simulink model "ES002A_McuDiagc"  (R2013b)
settings: Solver=FixedStepDiscrete  SolverMode=SingleTasking  StartTime=0.0  StopTime=1  FixedStep=0.000125  RelTol=1e-3
values from neighbouring files (symbols this model uses):
  dMcuDiagcFastLoopCntrMax = DataDict.Display    [ES002A_McuDiagc_DataDict.m]
  dMcuDiagcFastLoopCntrMin = DataDict.Display    [ES002A_McuDiagc_DataDict.m]
  dMcuDiagcLoopCntr2MilliSecMotCtrlDif = DataDict.Display    [ES002A_McuDiagc_DataDict.m]
  FastLoopCntr = DataDict.IpSignal    [ES002A_McuDiagc_DataDict.m]
  FASTLOOPCNTRMAX_CNT_U08 = DataDict.Constant    [ES002A_McuDiagc_DataDict.m]
  FASTLOOPCNTRMIN_CNT_U08 = DataDict.Constant    [ES002A_McuDiagc_DataDict.m]
  FastLoopCntrPrev = DataDict.PIM    [ES002A_McuDiagc_DataDict.m]
  LOOPCNTR2MILLISECMOTCTRLCOMPPRM_CNT_U08 = DataDict.Constant    [ES002A_McuDiagc_DataDict.m]
  LOSSMOTCTRLLOOPPRM_CNT_U08 = DataDict.Constant    [ES002A_McuDiagc_DataDict.m]
  McuDiagc2MilliSecCntrCompThd = DataDict.Calibration    [ES002A_McuDiagc_DataDict.m]
  McuDiagcFlt = DataDict.NTC    [ES002A_McuDiagc_DataDict.m]
  McuDiagcFltFailStep = DataDict.Calibration    [ES002A_McuDiagc_DataDict.m]
  McuDiagcFltPassStep = DataDict.Calibration    [ES002A_McuDiagc_DataDict.m]
  MOTCTRLDIAGCINITDLY_CNT_U08 = DataDict.Constant    [ES002A_McuDiagc_DataDict.m]
undefined symbols (not defined in the file or in its folder): NtcSts1, sigbuilder_block
libraries: simulink x10, NxtrMax x1, NxtrMin x1
(part 1 of 2)
settings Model: RequirementInfo="{}  %GIDa_ca294f38_ed7c_4fb9_8c54_f4d56271bfc7"  ModifiedHistory=Rev 008: Updated model to Matlab 2013B, added comments to show requirement linkage  Creator=nz3zln  LastModifiedBy=wzvp6q
settings SolverCC: AutoInsertRateTranBlk=on  InsertRTBMode=Always
settings DataIOCC: LimitDataPoints=off  SaveFormat=Structure  ReturnWorkspaceOutputs=on
settings OptimizationCC: BlockReduction=off  InlineParams=on  ZeroExternalMemoryAtStartup=off  ZeroInternalMemoryAtStartup=off  OptimizeModelRefInitCode=on  LifeSpan=1
settings DebuggingCC: SignalInfNanChecking=error  SignalRangeChecking=warning  UnderspecifiedInitializationDetection=Simplified  SolverPrmCheckMsg=error  InheritedTsInSrcMsg=error  DiscreteInheritContinuousMsg=error  SingleTaskRateTransMsg=error  TasksWithSamePriorityMsg=error  SigSpecEnsureSampleTimeMsg=error  CheckMatrixSingularityMsg=error  ParameterUnderflowMsg=error  ParameterPrecisionLossMsg=error  ParameterTunabilityLossMsg=error  FixptConstUnderflowMsg=warning  FixptConstOverflowMsg=warning  VectorMatrixConversionMsg=error  SignalLabelMismatchMsg=error  UnconnectedInputMsg=error  UnconnectedOutputMsg=error  UnconnectedLineMsg=error  SFcnCompatibilityMsg=error  UniqueDataStoreMsg=warning  BusObjectLabelMismatch=error  RootOutportRequireBusObject=error  AssertControl=DisableAll  ModelReferenceIOMsg=error  ModelReferenceVersionMismatchMessage=warning  ModelReferenceIOMismatchMessage=error  ModelReferenceCSMismatchMessage=warning  ModelReferenceDataLoggingMessage=error  StateNameClashWarn=warning  StrictBusMsg=ErrorOnBusTreatedAsVector  NonBusSignalsTreatedAsBus=error  SFUnexpectedBacktrackingDiag=error  SFInvalidInputDataAccessInChartInitDiag=error  SFNoUnconditionalDefaultTransitionDiag=error  SFTransitionOutsideNaturalParentDiag=error  SFUnconditionalTransitionShadowingDiag=error  SFUndirectedBroadcastEventsDiag=error
settings ModelReferenceCC: ModelReferenceNumInstancesAllowed=Single
settings RTWCC: SystemTargetFile=autosar.tlc  GenCodeOnly=on  TemplateMakefile=ert_default_tmf  Description=AUTOSAR  GenerateReport=on  ProcessScript=autosar_make_rtw_hook  LaunchReport=on
settings CodeAppCC: GenerateComments=off  IgnoreCustomStorageClasses=off  CustomSymbolStrType=$N$R$M  CustomSymbolStrBlkIO=$N$M  SimulinkBlockComments=off
settings STFCustomTargetCC: ParMdlRefBuildCompliant=on  CompOptLevelCompliant=on  IncludeMdlTerminateFcn=off  CombineOutputUpdateFcns=on  SuppressErrorStatus=on  ERTFirstTimeCompliant=on  ERTCustomFileBanners=on  SupportNonFinite=off  SupportComplex=off  SupportContinuousTime=off  SupportNonInlinedSFcns=off  MATLABClassNameForMDSCustomization=Simulink.SoftwareTarget.ERTCustomization  AutosarCompliant=on  GRTInterface=off  SystemTargetFile=autosar.tlc
settings ERTTargetCC: CodeReplacementLibrary=ANSI_C  ConcurrentExecutionCompliant=off  IncludeMdlTerminateFcn=off  SuppressErrorStatus=on  SupportNonFinite=off  SupportComplex=off  ModelStepFunctionPrototypeControlCompliant=off  CPPClassGenCompliant=off  AutosarCompliant=on  InlinedParameterPlacement=NonHierarchical  ERTCustomFileTemplate=example_file_process.tlc  EnableUserReplacementTypes=on

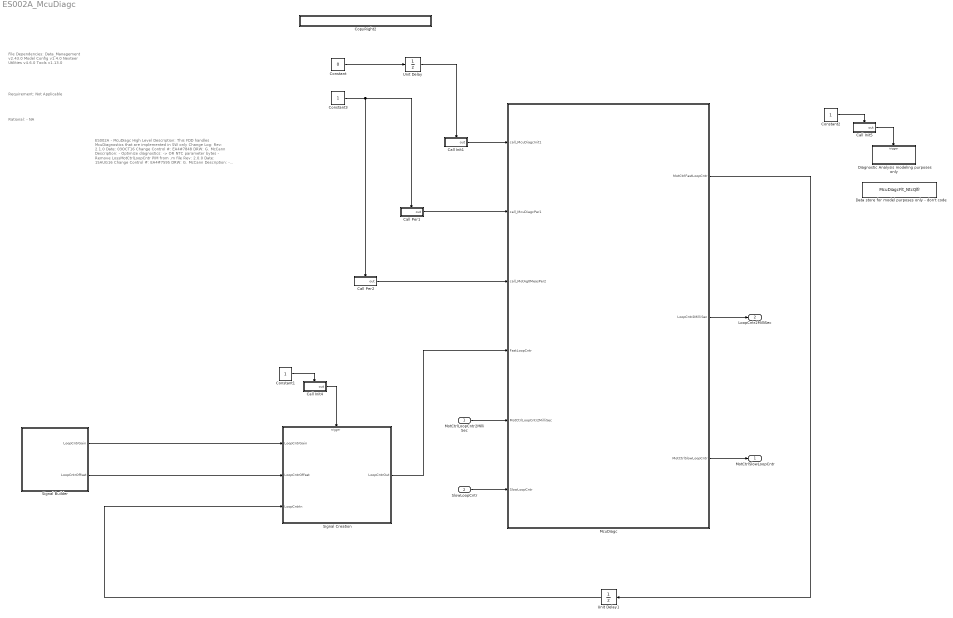
== system ES002A_McuDiagc ==
  note: ES002A - McuDiagc
      | High Level Description:
      | This FDD handles McuDiagnostics that are implemented in SW only
      |
      | Change Log:
      |
      | Rev: 2.1.0
      | Date: 03OCT16
      | Change Control #: EA4#7848
      | DRW: G. McCann
      | Description:
      | - Optimize diagnostics:
      |    -> OR NTC parameter bytes
      | - Remove LossMotCtrlLoopCntr PIM from .m file
      |
      | Rev: 2.0.0
      | Date: 15AUG16
      | Change Control #: EA4#7595
      | DRW: G. McCann
      | Description:
      | - Optimize diagnostics:
      |    -> Remove Per3 and associated IRVs
      |    -> Move relevant diagnostics that were in Per3 to Per2
      | - M file change: Update "ReadIn" property of input signals
      | "MotCtrlLoopCntr2MilliSec" and "SlowLoopCntr"
      |
      | Rev: 1.5.0
      | Date: 28JUN16
      | Change Control #: ICR-EA4#6452
      | DRW: G. McCann
      | Description:
      | -  Add IRVs for passing FastLoopCntrDiagcCfgd from Per2 to Per3.
      | This will allow a constant number of 2ms loops to pass before doing
      | the initial fault determination in Per3.
      | - Add IRV to pass LossMotCtrlLoopCntr from Per2 to Per3.  This
      | corrects an issue with the previous revision in which the same PIM
      | was being used in two different periodic functions.
      |
      | Rev: 1.4.0
      | Date: 15JUN16
      | Change Control #: ICR-EA4#6157
      | DRW: G. McCann
      | Description:
      | -  Add diagnostic check to ensure the MotCtrl ISR is
      | receiving information from the 2ms periodic.
      |
      | Rev: 1.3.0
      | Date: 07JUN16
      | Change Control #: ICR-EA4#6089
      | DRW: K. Patel
      | Description:
      | - ISO Debounce logic Added for NTC 2B
      |
      | Rev: 1.2.0
      | Date: 09MAY16
      | Change Control #: ICR-EA4#5733
      | DRW: G. McCann
      | Description:
      | - Add conditional to McuDiagcPer2 to allow a constant number
      | of 2ms loops to pass before doing the initial fault determination
      |
      | Rev: 1.0.0
      | Date: 23MAR16
      | Change Control #: ICR-EA4#49112
      | DRW: J. Erlenbeck
      | Description:
      | - Initial Release
  note: File Dependencies:
      | Data_Management v2.43.0
      | Model Config v1.4.0
      | Nexteer Utilities v4.6.0
      | Tools v1.13.0
  note: Requirement:
      | Not Applicable
  note: Rational:
      | - NA
  MotCtrlLoopCntr2MilliSec : Inport  RequirementInfo={} %GIDa_ea001b4b_5ccc_4bc9_bc0a_5435325e31ab  OutDataTypeStr=uint16
  SlowLoopCntr : Inport  Port=2  OutDataTypeStr=uint16
  Call Init1 : Subsystem  TreatAsAtomicUnit=on
  Call Init4 : Subsystem  TreatAsAtomicUnit=on
  Call Init5 : Subsystem  TreatAsAtomicUnit=on
  Call Per1 : Subsystem  TreatAsAtomicUnit=on
  Call Per2 : Subsystem  TreatAsAtomicUnit=on
  Constant : Constant  Value=0  OutDataTypeStr=uint8
  Constant1 : Constant  OutDataTypeStr=int8
  Constant2 : Constant  OutDataTypeStr=int8
  Constant3 : Constant  OutDataTypeStr=int8
  CopyRight2 : Subsystem  Description=|  mask(Copyright Information){none=on}
      | Copyright info block.                                               
      |                                                                     
      | Place copyright information at the top of every subsystem in design.
      mask prompts: none "No parameters"
      mask help: Place copyright information at the top of every subsystem in design.
      mask Display:
      | NxtrConf = 'Nexteer Confidential';
      | 
      | sys = bdroot; %handle for the current model ("system")
      | first = get_param(sys,'Created');
      | first = first(end-3:end);  %year is last four digits
      | 
      | last = get_param(sys,'LastModifiedDate');
      | if isempty(last)
      |     last = datestr(now,'yyyy');
      | else
      |     last = last(end-3:end);
      | end
      | 
      | if strcmp(first,last)
      |     fprintf('%s -- Copyright %s Nexteer',NxtrConf,first)
      | else
      |     fprintf('%s -- %s%s- %s Nexteer',NxtrConf,char(169),first,last)
      | end
  Data store for model purposes only - don't code : DataStoreMemory  DataStoreName=McuDiagcFlt_NtcQlfr
  Diagnostic Analysis modeling purposes only : Subsystem  TreatAsAtomicUnit=on
  McuDiagc : Subsystem
  Signal Builder : Subsystem  Tag=STV Subsys  LoadFcn=sigbuilder_block('load');  StartFcn=sigbuilder_block('start');  StopFcn=sigbuilder_block('stop');  ClipboardFcn=sigbuilder_block('clipboard');  mask(Sigbuilder block){}
      mask help: Simulink:masks:SigbuilderBlock_MD
      mask init:
      | if ~strcmp(get_param(bdroot(gcbh),'SimulationStatus'),'stopped') tuvar = sigbuilder_block('maskInit'); end
      settings: CopyFcn=sigbuilder_block('copy');  DeleteFcn=sigbuilder_block('delete');  ModelCloseFcn=sigbuilder_block('modelClose');  PreSaveFcn=sigbuilder_block('preSave');  PauseFcn=sigbuilder_block('pause');  ContinueFcn=sigbuilder_block('continue');  NameChangeFcn=sigbuilder_block('namechange');  OpenFcn=sigbuilder_block('open',[6 6 1012.5 507 ]);  CloseFcn=sigbuilder_block('close');
      mask Display: plot(0, 0, 100, 100,[2, 2, 32, 32, 2], [68, 8, 8, 68, 68],[32, 2], [38, 38], [32, 19, 2],[53, 60, 44], [32, 17, 17, 2],[16, 16, 31, 31]);txt = getActiveGroup(gcbh);text(2, 100, txt,'verticalAlignment', 'top');
  Signal Creation : Subsystem
  Unit Delay : UnitDelay  InitialCondition=1  SampleTime=-1
  Unit Delay1 : UnitDelay  SampleTime=-1
  MotCtrlSlowLoopCntr : Outport
  LoopCntr2MilliSec : Outport  Port=2
  wires:
  Constant/1 -> Unit Delay/1
  Unit Delay/1 -> Call Init1/Enable
  Constant3/1 -> Call Per1/Enable, Call Per2/Enable
  Call Init1/1(out) -> McuDiagc/1(call_McuDiagcInit1)
  Call Per1/1(out) -> McuDiagc/2(call_McuDiagcPer1)
  Call Per2/1(out) -> McuDiagc/3(call_MotAg0MeasPer2)
  Unit Delay1/1 -> Signal Creation/3(LoopCntrIn)
  Constant1/1 -> Call Init4/Enable
  Call Init4/1(out) -> Signal Creation/Trigger
  Signal Builder/1(LoopCntrGain) -> Signal Creation/1(LoopCntrGain)
  Signal Builder/2(LoopCntrOffset) -> Signal Creation/2(LoopCntrOffset)
  Signal Creation/1(LoopCntrOut) -> McuDiagc/4(FastLoopCntr)
  McuDiagc/1(MotCtrlFastLoopCntr) -> Unit Delay1/1
  Constant2/1 -> Call Init5/Enable
  Call Init5/1(out) -> Diagnostic Analysis modeling purposes only/Trigger
  McuDiagc/3(MotCtrlSlowLoopCntr) -> MotCtrlSlowLoopCntr/1
  McuDiagc/2(LoopCntr2MilliSec) -> LoopCntr2MilliSec/1
  MotCtrlLoopCntr2MilliSec/1 -> McuDiagc/5(MotCtrlLoopCntr2MilliSec)
  SlowLoopCntr/1 -> McuDiagc/6(SlowLoopCntr)

== system ES002A_McuDiagc/Call Init1 ==
  Enable : EnablePort
  Function Call Trigger : simulink/Ports & Subsystems/Function-Call Generator  RequirementInfo={} %GIDa_ff755a2e_49d1_45f7_8591_3ce0ef475338  sample_time=0.002  numberOfIterations=1
  out : Outport
  wires:
  Function Call Trigger/1 -> out/1

== system ES002A_McuDiagc/Call Init4 ==
  Enable : EnablePort
  Function Call Trigger : simulink/Ports & Subsystems/Function-Call Generator  RequirementInfo={} %GIDa_6dd05ab1_f91b_4d7a_a0ec_1170d213fa7b  sample_time=0.000125  numberOfIterations=1
  out : Outport
  wires:
  Function Call Trigger/1 -> out/1

== system ES002A_McuDiagc/Call Init5 ==
  Enable : EnablePort
  Function Call Trigger : simulink/Ports & Subsystems/Function-Call Generator  RequirementInfo={} %GIDa_75efe8f1_d27f_4e45_b6fa_68d4c3186d57  sample_time=0.002  numberOfIterations=1
  out : Outport
  wires:
  Function Call Trigger/1 -> out/1

== system ES002A_McuDiagc/Call Per1 ==
  Enable : EnablePort
  Function Call Trigger : simulink/Ports & Subsystems/Function-Call Generator  RequirementInfo={} %GIDa_6dd05ab1_f91b_4d7a_a0ec_1170d213fa7b  sample_time=0.000125  numberOfIterations=1
  out : Outport
  wires:
  Function Call Trigger/1 -> out/1

== system ES002A_McuDiagc/Call Per2 ==
  Enable : EnablePort
  Function Call Trigger : simulink/Ports & Subsystems/Function-Call Generator  RequirementInfo={} %GIDa_9bd65ccd_39f3_4e48_9d09_4984d13bbcbb  sample_time=0.002  numberOfIterations=1
  out : Outport
  wires:
  Function Call Trigger/1 -> out/1

== system ES002A_McuDiagc/CopyRight2 ==

== system ES002A_McuDiagc/Diagnostic Analysis modeling purposes only ==
  function : TriggerPort  TriggerType=function-call
  CopyRight2 : Subsystem  Description=|  mask(Copyright Information){none=on}
      | Copyright info block.                                               
      |                                                                     
      | Place copyright information at the top of every subsystem in design.
      mask prompts: none "No parameters"
      mask help: Place copyright information at the top of every subsystem in design.
      mask Display:
      | NxtrConf = 'Nexteer Confidential';
      | 
      | sys = bdroot; %handle for the current model ("system")
      | first = get_param(sys,'Created');
      | first = first(end-3:end);  %year is last four digits
      | 
      | last = get_param(sys,'LastModifiedDate');
      | if isempty(last)
      |     last = datestr(now,'yyyy');
      | else
      |     last = last(end-3:end);
      | end
      | 
      | if strcmp(first,last)
      |     fprintf('%s -- Copyright %s Nexteer',NxtrConf,first)
      | else
      |     fprintf('%s -- %s%s- %s Nexteer',NxtrConf,char(169),first,last)
      | end
  Data Store Read1 : DataStoreRead  DataStoreName=McuDiagcFlt_NtcQlfr
  Scope : Scope
  wires:
  Data Store Read1/1 -> Scope/1

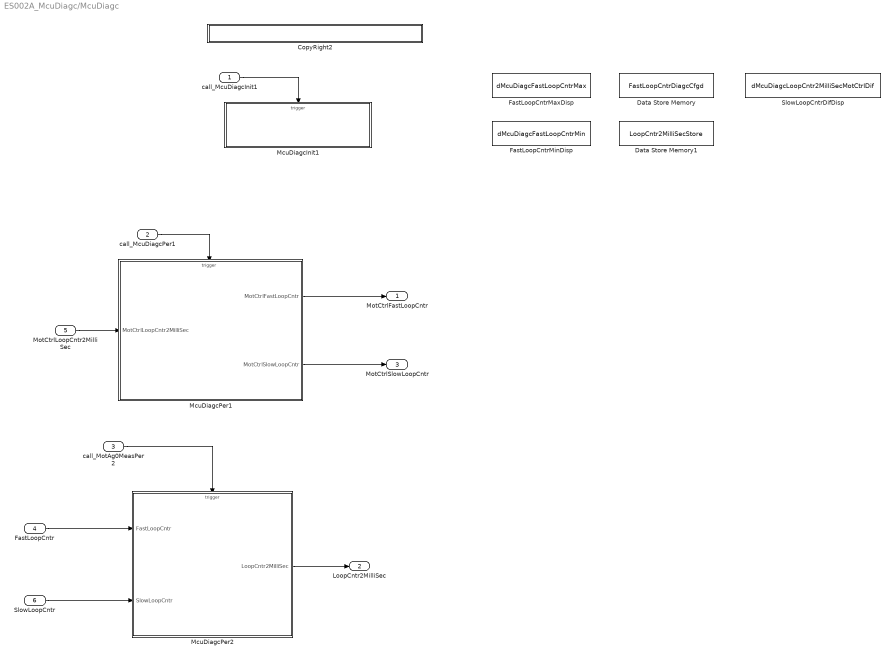
== system ES002A_McuDiagc/McuDiagc ==
  call_McuDiagcInit1 : Inport  RequirementInfo={} %GIDa_18b4b7a7_d8ff_42fd_afd9_8fbc558fb7ae
  call_McuDiagcPer1 : Inport  RequirementInfo={} %GIDa_8c56c68f_1996_47ee_bda4_35b4dc112bcf  Port=2
  call_MotAg0MeasPer2 : Inport  RequirementInfo={} %GIDa_7b28921c_189e_46dc_b03b_f7509365a7f9  Port=3
  FastLoopCntr : Inport  Port=4
  MotCtrlLoopCntr2MilliSec : Inport  RequirementInfo={} %GIDa_9cfa8093_7f6c_44dd_ac23_c949c563b3b4  Port=5
  SlowLoopCntr : Inport  Port=6
  CopyRight2 : Subsystem  Description=|  mask(Copyright Information){none=on}
      | Copyright info block.                                               
      |                                                                     
      | Place copyright information at the top of every subsystem in design.
      mask prompts: none "No parameters"
      mask help: Place copyright information at the top of every subsystem in design.
      mask Display:
      | NxtrConf = 'Nexteer Confidential';
      | 
      | sys = bdroot; %handle for the current model ("system")
      | first = get_param(sys,'Created');
      | first = first(end-3:end);  %year is last four digits
      | 
      | last = get_param(sys,'LastModifiedDate');
      | if isempty(last)
      |     last = datestr(now,'yyyy');
      | else
      |     last = last(end-3:end);
      | end
      | 
      | if strcmp(first,last)
      |     fprintf('%s -- Copyright %s Nexteer',NxtrConf,first)
      | else
      |     fprintf('%s -- %s%s- %s Nexteer',NxtrConf,char(169),first,last)
      | end
  Data Store Memory : DataStoreMemory  DataStoreName=FastLoopCntrDiagcCfgd  OutDataTypeStr=uint8  StateMustResolveToSignalObject=on
  Data Store Memory1 : DataStoreMemory  DataStoreName=LoopCntr2MilliSecStore  OutDataTypeStr=uint16  StateMustResolveToSignalObject=on
  FastLoopCntrMaxDisp : DataStoreMemory  DataStoreName=dMcuDiagcFastLoopCntrMax  StateMustResolveToSignalObject=on
  FastLoopCntrMinDisp : DataStoreMemory  DataStoreName=dMcuDiagcFastLoopCntrMin  StateMustResolveToSignalObject=on
  McuDiagcInit1 : Subsystem
  McuDiagcPer1 : Subsystem  RequirementInfo="{'linktype_rmi_doors' '00010239 (/ESG Group/FDD Module Requirements/EA4 Specific/ES002A_McuDiagc)' '#ES002A_15' 'true' 'REQ:  ES002A_15' '' } %GIDa_1a0e9409_eaa0_4ab7_bf19_c7a428015c57"  TreatAsAtomicUnit=on
  McuDiagcPer2 : Subsystem  RequirementInfo="{'linktype_rmi_doors' '00010239 (/ESG Group/FDD Module Requirements/EA4 Specific/ES002A_McuDiagc)' '#ES002A_15' 'true' 'REQ:  ES002A_15' '' } %GIDa_200460cd_1c5a_4721_859a_3560e07697e4"  TreatAsAtomicUnit=on
  SlowLoopCntrDifDisp : DataStoreMemory  DataStoreName=dMcuDiagcLoopCntr2MilliSecMotCtrlDif  OutDataTypeStr=uint16  StateMustResolveToSignalObject=on
  MotCtrlFastLoopCntr : Outport
  LoopCntr2MilliSec : Outport  Port=2
  MotCtrlSlowLoopCntr : Outport  Port=3
  wires:
  call_McuDiagcInit1/1 -> McuDiagcInit1/Trigger
  call_McuDiagcPer1/1 -> McuDiagcPer1/Trigger
  call_MotAg0MeasPer2/1 -> McuDiagcPer2/Trigger
  FastLoopCntr/1 -> McuDiagcPer2/1(FastLoopCntr)
  McuDiagcPer1/1(MotCtrlFastLoopCntr) -> MotCtrlFastLoopCntr/1
  McuDiagcPer1/2(MotCtrlSlowLoopCntr) -> MotCtrlSlowLoopCntr/1
  MotCtrlLoopCntr2MilliSec/1 -> McuDiagcPer1/1(MotCtrlLoopCntr2MilliSec)
  McuDiagcPer2/1(LoopCntr2MilliSec) -> LoopCntr2MilliSec/1
  SlowLoopCntr/1 -> McuDiagcPer2/2(SlowLoopCntr)

== system ES002A_McuDiagc/Signal Builder ==
  Demux : Demux  Tag=STV Demux  Outputs=2
  FromWs : FromWorkspace  Tag=STV FromWs  VariableName=tuvar  SampleTime=0
      SigBuilderData=|
      | common.afterFinalStr = 'Extrapolate'
      | common.sampleTime = 0
      | dataSet.timeRange = [0 10]
      | dataSet.name = 'Group 1'
      | sbobj.Groups.Name = 'Group 1'
      | sbobj.Groups.Signals(1).Name = 'LoopCntrGain'
      | sbobj.Groups.Signals(1).XData = [0 7.56 7.7 10]
      | sbobj.Groups.Signals(1).YData = [1 1 1 1]
      | sbobj.Groups.Signals(2).Name = 'LoopCntrOffset'
      | sbobj.Groups.Signals(2).XData = [0 7.675 7.675 9.494 9.494 10]
      | sbobj.Groups.Signals(2).YData = [0 0 100 100 0 0]
  LoopCntrGain : Outport  Tag=STV Outport
  LoopCntrOffset : Outport  Tag=STV Outport  Port=2
  wires:
  FromWs/1 -> Demux/1
  Demux/1 -> LoopCntrGain/1
  Demux/2 -> LoopCntrOffset/1

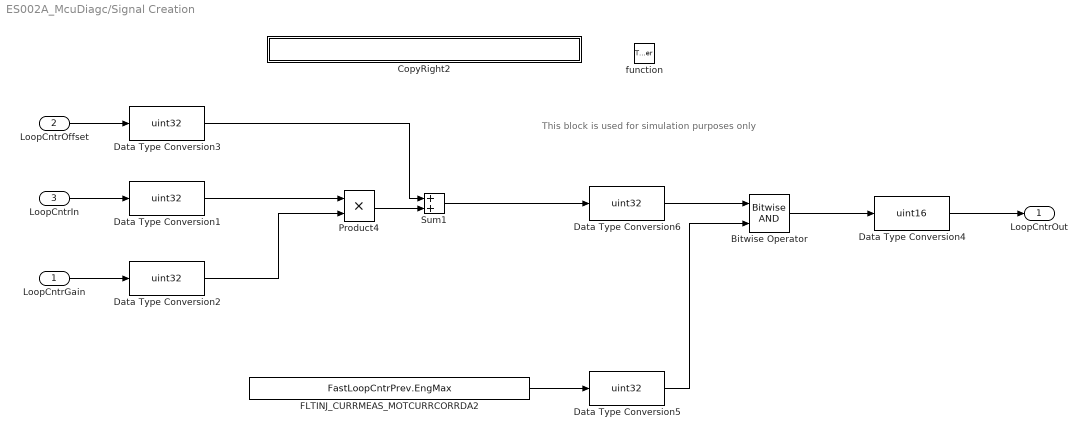
== system ES002A_McuDiagc/Signal Creation ==
  note: This block is used for simulation purposes only
  LoopCntrGain : Inport  RequirementInfo={} %GIDa_46ffa422_a9f2_4bcd_a096_e28769753b36
  LoopCntrOffset : Inport  RequirementInfo={} %GIDa_0564dd14_44e0_4b25_a7ea_7ef64c704b65  Port=2
  LoopCntrIn : Inport  RequirementInfo={} %GIDa_3b8fba3c_7125_490c_a301_802e8993f682  Port=3
  function : TriggerPort  TriggerType=function-call
  Bitwise Operator : simulink/Logic and Bit Operations/Bitwise Operator  logicop=AND  UseBitMask=off  NumInputPorts=2  BitMask=bin2dec('11011001')  BitMaskRealWorld=Stored Integer
  CopyRight2 : Subsystem  Description=|  mask(Copyright Information){none=on}
      | Copyright info block.                                               
      |                                                                     
      | Place copyright information at the top of every subsystem in design.
      mask prompts: none "No parameters"
      mask help: Place copyright information at the top of every subsystem in design.
      mask Display:
      | NxtrConf = 'Nexteer Confidential';
      | 
      | sys = bdroot; %handle for the current model ("system")
      | first = get_param(sys,'Created');
      | first = first(end-3:end);  %year is last four digits
      | 
      | last = get_param(sys,'LastModifiedDate');
      | if isempty(last)
      |     last = datestr(now,'yyyy');
      | else
      |     last = last(end-3:end);
      | end
      | 
      | if strcmp(first,last)
      |     fprintf('%s -- Copyright %s Nexteer',NxtrConf,first)
      | else
      |     fprintf('%s -- %s%s- %s Nexteer',NxtrConf,char(169),first,last)
      | end
  Data Type Conversion{1..3,5..6} (5 alike) : DataTypeConversion  OutMin=0  OutMax=2^32-1  OutDataTypeStr=uint32
  Data Type Conversion4 : DataTypeConversion  OutDataTypeStr=uint16
  FLTINJ_CURRMEAS_MOTCURRCORRDA2 : Constant  Value=FastLoopCntrPrev.EngMax  OutDataTypeStr=uint32
  Product4 : Product
  Sum1 : Sum
  LoopCntrOut : Outport
  wires:
  LoopCntrGain/1 -> Data Type Conversion2/1
  LoopCntrIn/1 -> Data Type Conversion1/1
  Data Type Conversion3/1 -> Sum1/1
  Data Type Conversion1/1 -> Product4/1
  Data Type Conversion2/1 -> Product4/2
  LoopCntrOffset/1 -> Data Type Conversion3/1
  Product4/1 -> Sum1/2
  Sum1/1 -> Data Type Conversion6/1
  FLTINJ_CURRMEAS_MOTCURRCORRDA2/1 -> Data Type Conversion5/1
  Bitwise Operator/1 -> Data Type Conversion4/1
  Data Type Conversion4/1 -> LoopCntrOut/1
  Data Type Conversion5/1 -> Bitwise Operator/2
  Data Type Conversion6/1 -> Bitwise Operator/1

== system ES002A_McuDiagc/Diagnostic Analysis modeling purposes only/CopyRight2 ==

== system ES002A_McuDiagc/McuDiagc/CopyRight2 ==

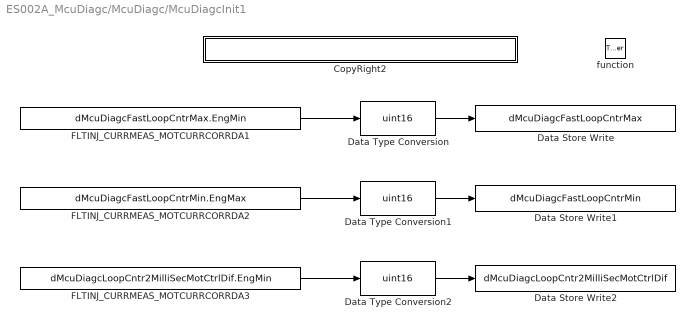
== system ES002A_McuDiagc/McuDiagc/McuDiagcInit1 ==
  function : TriggerPort  TriggerType=function-call
  CopyRight2 : Subsystem  Description=|  mask(Copyright Information){none=on}
      | Copyright info block.                                               
      |                                                                     
      | Place copyright information at the top of every subsystem in design.
      mask prompts: none "No parameters"
      mask help: Place copyright information at the top of every subsystem in design.
      mask Display:
      | NxtrConf = 'Nexteer Confidential';
      | 
      | sys = bdroot; %handle for the current model ("system")
      | first = get_param(sys,'Created');
      | first = first(end-3:end);  %year is last four digits
      | 
      | last = get_param(sys,'LastModifiedDate');
      | if isempty(last)
      |     last = datestr(now,'yyyy');
      | else
      |     last = last(end-3:end);
      | end
      | 
      | if strcmp(first,last)
      |     fprintf('%s -- Copyright %s Nexteer',NxtrConf,first)
      | else
      |     fprintf('%s -- %s%s- %s Nexteer',NxtrConf,char(169),first,last)
      | end
  Data Store Write : DataStoreWrite  DataStoreName=dMcuDiagcFastLoopCntrMax
  Data Store Write1 : DataStoreWrite  DataStoreName=dMcuDiagcFastLoopCntrMin
  Data Store Write2 : DataStoreWrite  DataStoreName=dMcuDiagcLoopCntr2MilliSecMotCtrlDif
  Data Type Conversion : DataTypeConversion  OutDataTypeStr=uint16
  Data Type Conversion1 : DataTypeConversion  OutDataTypeStr=uint16
  Data Type Conversion2 : DataTypeConversion  OutDataTypeStr=uint16
  FLTINJ_CURRMEAS_MOTCURRCORRDA1 : Constant  Value=dMcuDiagcFastLoopCntrMax.EngMin  OutDataTypeStr=uint32
  FLTINJ_CURRMEAS_MOTCURRCORRDA2 : Constant  Value=dMcuDiagcFastLoopCntrMin.EngMax  OutDataTypeStr=uint32
  FLTINJ_CURRMEAS_MOTCURRCORRDA3 : Constant  Value=dMcuDiagcLoopCntr2MilliSecMotCtrlDif.EngMin  OutDataTypeStr=uint32
  wires:
  FLTINJ_CURRMEAS_MOTCURRCORRDA1/1 -> Data Type Conversion/1
  Data Type Conversion/1 -> Data Store Write/1
  FLTINJ_CURRMEAS_MOTCURRCORRDA2/1 -> Data Type Conversion1/1
  Data Type Conversion1/1 -> Data Store Write1/1
  Data Type Conversion2/1 -> Data Store Write2/1
  FLTINJ_CURRMEAS_MOTCURRCORRDA3/1 -> Data Type Conversion2/1

== system ES002A_McuDiagc/McuDiagc/McuDiagcPer1 ==
  MotCtrlLoopCntr2MilliSec : Inport
  function : TriggerPort  TriggerType=function-call
  CopyRight2 : Subsystem  Description=|  mask(Copyright Information){none=on}
      | Copyright info block.                                               
      |                                                                     
      | Place copyright information at the top of every subsystem in design.
      mask prompts: none "No parameters"
      mask help: Place copyright information at the top of every subsystem in design.
      mask Display:
      | NxtrConf = 'Nexteer Confidential';
      | 
      | sys = bdroot; %handle for the current model ("system")
      | first = get_param(sys,'Created');
      | first = first(end-3:end);  %year is last four digits
      | 
      | last = get_param(sys,'LastModifiedDate');
      | if isempty(last)
      |     last = datestr(now,'yyyy');
      | else
      |     last = last(end-3:end);
      | end
      | 
      | if strcmp(first,last)
      |     fprintf('%s -- Copyright %s Nexteer',NxtrConf,first)
      | else
      |     fprintf('%s -- %s%s- %s Nexteer',NxtrConf,char(169),first,last)
      | end
  Increment ISR Based Accumulator : Subsystem  RequirementInfo="{'linktype_rmi_doors' '00010239 (/ESG Group/FDD Module Requirements/EA4 Specific/ES002A_McuDiagc)' '#ES002A_35' 'true' 'REQ:  ES002A_35' '' ; 'linktype_rmi_doors' '00010239 (/ESG Group/FDD Module Requirements/EA4 Specific/ES002A_McuDiagc)' '#ES002A_76' 'true' 'REQ:ES002A_76' '' } %GIDa_f7d07956_e6e9_4f91_b80a_5fc94a64cb9d"  TreatAsAtomicUnit=on
  MotCtrlFastLoopCntr : Outport
  MotCtrlSlowLoopCntr : Outport  Port=2
  wires:
  Increment ISR Based Accumulator/1(MotCtrlFastLoopCntr) -> MotCtrlFastLoopCntr/1
  MotCtrlLoopCntr2MilliSec/1 -> MotCtrlSlowLoopCntr/1

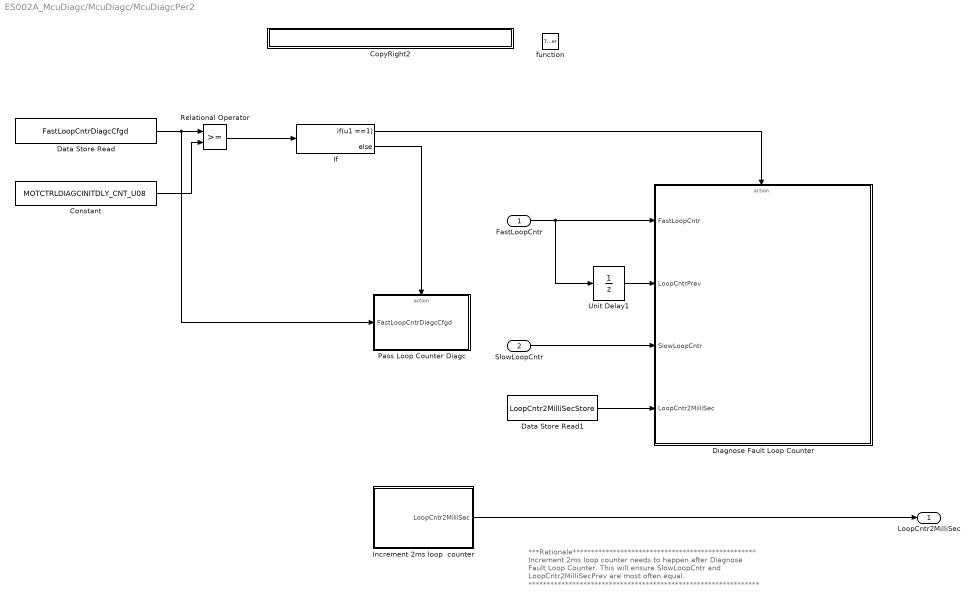
== system ES002A_McuDiagc/McuDiagc/McuDiagcPer2 ==
  note: ***Rationale**************************************************
      | Increment 2ms loop counter needs to happen after
      | Diagnose Fault Loop Counter.
      | This will ensure SlowLoopCntr and LoopCntr2MilliSecPrev
      | are most often equal.
      | ***************************************************************
  FastLoopCntr : Inport
  SlowLoopCntr : Inport  Port=2
  function : TriggerPort  TriggerType=function-call
  Constant : Constant  Value=MOTCTRLDIAGCINITDLY_CNT_U08  OutDataTypeStr=uint8
  CopyRight2 : Subsystem  Description=|  mask(Copyright Information){none=on}
      | Copyright info block.                                               
      |                                                                     
      | Place copyright information at the top of every subsystem in design.
      mask prompts: none "No parameters"
      mask help: Place copyright information at the top of every subsystem in design.
      mask Display:
      | NxtrConf = 'Nexteer Confidential';
      | 
      | sys = bdroot; %handle for the current model ("system")
      | first = get_param(sys,'Created');
      | first = first(end-3:end);  %year is last four digits
      | 
      | last = get_param(sys,'LastModifiedDate');
      | if isempty(last)
      |     last = datestr(now,'yyyy');
      | else
      |     last = last(end-3:end);
      | end
      | 
      | if strcmp(first,last)
      |     fprintf('%s -- Copyright %s Nexteer',NxtrConf,first)
      | else
      |     fprintf('%s -- %s%s- %s Nexteer',NxtrConf,char(169),first,last)
      | end
  Data Store Read : DataStoreRead  DataStoreName=FastLoopCntrDiagcCfgd
  Data Store Read1 : DataStoreRead  DataStoreName=LoopCntr2MilliSecStore
  Diagnose Fault Loop Counter : Subsystem  Priority=10  TreatAsAtomicUnit=on
      settings: AttributesFormatString=Priority: %<Priority>
  If : If  RequirementInfo="{'linktype_rmi_doors' '00010239 (/ESG Group/FDD Module Requirements/EA4 Specific/ES002A_McuDiagc)' '#ES002A_25' 'true' 'REQ:  ES002A_25' '' } %GIDa_92b02519_41af_445c_925f_66c2deedfe4e"  IfExpression=u1 ==1
  Increment 2ms loop  counter : Subsystem  RequirementInfo={'linktype_rmi_doors' '00010239 (/ESG Group/FDD Module Requirements/EA4 Specific/ES002A_McuDiagc)' '#ES002A_72' 'true' 'REQ:ES002A_72' '' ; 'linktype_rmi_doors' '00010239 (/ESG Group/FDD Module Requirements/EA4 Specific/ES002A_McuDiagc)' '#ES002A_77' 'true' 'REQ:ES002A_77' '' } %GIDa_5de7e1bd_4d4c_467c_aadf_b7bb5ec147fa  Priority=20
      settings: AttributesFormatString=Priority: %<Priority>
  Pass Loop Counter Diagc : Subsystem  TreatAsAtomicUnit=on
  Relational Operator : RelationalOperator  OutDataTypeStr=boolean
  Unit Delay1 : UnitDelay  SampleTime=-1  StateName=LoopCntrPrev  StateMustResolveToSignalObject=on
      settings: AttributesFormatString=|
      | State Variable:
      | %<StateName>
  LoopCntr2MilliSec : Outport
  wires:
  FastLoopCntr/1 -> Diagnose Fault Loop Counter/1(FastLoopCntr), Unit Delay1/1
  Unit Delay1/1 -> Diagnose Fault Loop Counter/2(LoopCntrPrev)
  If/1 -> Diagnose Fault Loop Counter/Action
  If/2 -> Pass Loop Counter Diagc/Action
  Constant/1 -> Relational Operator/2
  Data Store Read/1 -> Pass Loop Counter Diagc/1(FastLoopCntrDiagcCfgd), Relational Operator/1
  Relational Operator/1 -> If/1
  Increment 2ms loop  counter/1(LoopCntr2MilliSec) -> LoopCntr2MilliSec/1
  SlowLoopCntr/1 -> Diagnose Fault Loop Counter/3(SlowLoopCntr)
  Data Store Read1/1 -> Diagnose Fault Loop Counter/4(LoopCntr2MilliSec)

== system ES002A_McuDiagc/Signal Creation/CopyRight2 ==

== system ES002A_McuDiagc/McuDiagc/McuDiagcInit1/CopyRight2 ==

== system ES002A_McuDiagc/McuDiagc/McuDiagcPer1/CopyRight2 ==

== system ES002A_McuDiagc/McuDiagc/McuDiagcPer1/Increment ISR Based Accumulator ==
  note: ******  Note that these operations may be
      | optimized in the code.  The purpose of this code
      | is to create a counter that increment every loop and
      | rolls over when the counter reaches 65535.
  Bias : Bias  Bias=1.0
  Bitwise Operator : simulink/Logic and Bit Operations/Bitwise Operator  logicop=AND  UseBitMask=off  NumInputPorts=2  BitMask=bin2dec('11011001')  BitMaskRealWorld=Stored Integer
  CopyRight2 : Subsystem  Description=|  mask(Copyright Information){none=on}
      | Copyright info block.                                               
      |                                                                     
      | Place copyright information at the top of every subsystem in design.
      mask prompts: none "No parameters"
      mask help: Place copyright information at the top of every subsystem in design.
      mask Display:
      | NxtrConf = 'Nexteer Confidential';
      | 
      | sys = bdroot; %handle for the current model ("system")
      | first = get_param(sys,'Created');
      | first = first(end-3:end);  %year is last four digits
      | 
      | last = get_param(sys,'LastModifiedDate');
      | if isempty(last)
      |     last = datestr(now,'yyyy');
      | else
      |     last = last(end-3:end);
      | end
      | 
      | if strcmp(first,last)
      |     fprintf('%s -- Copyright %s Nexteer',NxtrConf,first)
      | else
      |     fprintf('%s -- %s%s- %s Nexteer',NxtrConf,char(169),first,last)
      | end
  Data Type Conversion : DataTypeConversion  OutDataTypeStr=uint32
  Data Type Conversion1 : DataTypeConversion  OutDataTypeStr=uint16
  FLTINJ_CURRMEAS_MOTCURRCORRDA2 : Constant  Value=FastLoopCntrPrev.EngMax  OutDataTypeStr=uint32
  Unit Delay : UnitDelay  SampleTime=-1  StateName=FastLoopCntrPrev  StateMustResolveToSignalObject=on
      settings: AttributesFormatString=|
      | State Variable:
      | %<StateName>
  MotCtrlFastLoopCntr : Outport
  wires:
  Unit Delay/1 -> Data Type Conversion/1
  Data Type Conversion/1 -> Bias/1
  Bias/1 -> Bitwise Operator/1
  FLTINJ_CURRMEAS_MOTCURRCORRDA2/1 -> Bitwise Operator/2
  Bitwise Operator/1 -> Data Type Conversion1/1
  Data Type Conversion1/1 -> MotCtrlFastLoopCntr/1, Unit Delay/1

== system ES002A_McuDiagc/McuDiagc/McuDiagcPer2/CopyRight2 ==

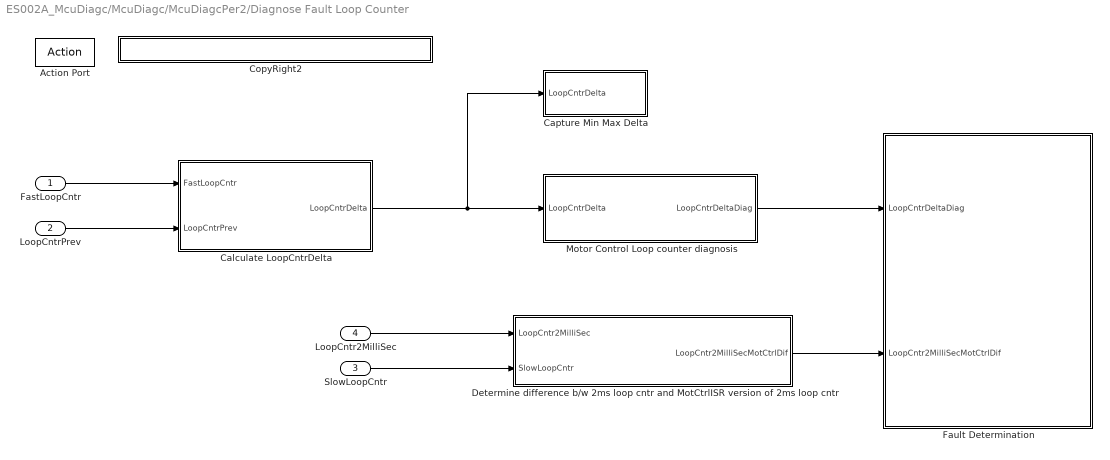
== system ES002A_McuDiagc/McuDiagc/McuDiagcPer2/Diagnose Fault Loop Counter ==
  FastLoopCntr : Inport
  LoopCntrPrev : Inport  Port=2
  SlowLoopCntr : Inport  Port=3
  LoopCntr2MilliSec : Inport  Port=4
  Action Port : ActionPort  ActionType=then
  Calculate LoopCntrDelta : Subsystem  TreatAsAtomicUnit=on
  Capture Min Max Delta : Subsystem  TreatAsAtomicUnit=on
  CopyRight2 : Subsystem  Description=|  mask(Copyright Information){none=on}
      | Copyright info block.                                               
      |                                                                     
      | Place copyright information at the top of every subsystem in design.
      mask prompts: none "No parameters"
      mask help: Place copyright information at the top of every subsystem in design.
      mask Display:
      | NxtrConf = 'Nexteer Confidential';
      | 
      | sys = bdroot; %handle for the current model ("system")
      | first = get_param(sys,'Created');
      | first = first(end-3:end);  %year is last four digits
      | 
      | last = get_param(sys,'LastModifiedDate');
      | if isempty(last)
      |     last = datestr(now,'yyyy');
      | else
      |     last = last(end-3:end);
      | end
      | 
      | if strcmp(first,last)
      |     fprintf('%s -- Copyright %s Nexteer',NxtrConf,first)
      | else
      |     fprintf('%s -- %s%s- %s Nexteer',NxtrConf,char(169),first,last)
      | end
  Determine difference b/w 2ms loop cntr and MotCtrlISR version of 2ms loop cntr : Subsystem  RequirementInfo="{'linktype_rmi_doors' '00010239 (/ESG Group/FDD Module Requirements/EA4 Specific/ES002A_McuDiagc)' '#ES002A_75' 'true' 'REQ:  ES002A_75' '' } %GIDa_e4bb4a0a_d754_4298_81cf_0d6eaaf09216"  TreatAsAtomicUnit=on
  Fault Determination : Subsystem  TreatAsAtomicUnit=on
  Motor Control Loop counter diagnosis : Subsystem  TreatAsAtomicUnit=on
  wires:
  FastLoopCntr/1 -> Calculate LoopCntrDelta/1(FastLoopCntr)
  LoopCntrPrev/1 -> Calculate LoopCntrDelta/2(LoopCntrPrev)
  Calculate LoopCntrDelta/1(LoopCntrDelta) -> Motor Control Loop counter diagnosis/1(LoopCntrDelta), Capture Min Max Delta/1(LoopCntrDelta)
  LoopCntr2MilliSec/1 -> Determine difference b/w 2ms loop cntr and MotCtrlISR version of 2ms loop cntr/1(LoopCntr2MilliSec)
  SlowLoopCntr/1 -> Determine difference b/w 2ms loop cntr and MotCtrlISR version of 2ms loop cntr/2(SlowLoopCntr)
  Motor Control Loop counter diagnosis/1(LoopCntrDeltaDiag) -> Fault Determination/1(LoopCntrDeltaDiag)
  Determine difference b/w 2ms loop cntr and MotCtrlISR version of 2ms loop cntr/1(LoopCntr2MilliSecMotCtrlDif) -> Fault Determination/2(LoopCntr2MilliSecMotCtrlDif)

== system ES002A_McuDiagc/McuDiagc/McuDiagcPer2/Increment 2ms loop  counter ==
  Add : Sum  OutDataTypeStr=uint16
  Constant1 : Constant  OutDataTypeStr=uint16
  CopyRight2 : Subsystem  Description=|  mask(Copyright Information){none=on}
      | Copyright info block.                                               
      |                                                                     
      | Place copyright information at the top of every subsystem in design.
      mask prompts: none "No parameters"
      mask help: Place copyright information at the top of every subsystem in design.
      mask Display:
      | NxtrConf = 'Nexteer Confidential';
      | 
      | sys = bdroot; %handle for the current model ("system")
      | first = get_param(sys,'Created');
      | first = first(end-3:end);  %year is last four digits
      | 
      | last = get_param(sys,'LastModifiedDate');
      | if isempty(last)
      |     last = datestr(now,'yyyy');
      | else
      |     last = last(end-3:end);
      | end
      | 
      | if strcmp(first,last)
      |     fprintf('%s -- Copyright %s Nexteer',NxtrConf,first)
      | else
      |     fprintf('%s -- %s%s- %s Nexteer',NxtrConf,char(169),first,last)
      | end
  Data Store Read1 : DataStoreRead  DataStoreName=LoopCntr2MilliSecStore
  Data Store Write : DataStoreWrite  DataStoreName=LoopCntr2MilliSecStore
  LoopCntr2MilliSec : Outport
  wires:
  Data Store Read1/1 -> Add/1
  Constant1/1 -> Add/2
  Add/1 -> LoopCntr2MilliSec/1, Data Store Write/1

== system ES002A_McuDiagc/McuDiagc/McuDiagcPer2/Pass Loop Counter Diagc ==
  FastLoopCntrDiagcCfgd : Inport
  Action Port : ActionPort  ActionType=else
  Add : Sum  OutDataTypeStr=uint8
  Constant : Constant  OutDataTypeStr=uint8
  CopyRight2 : Subsystem  Description=|  mask(Copyright Information){none=on}
      | Copyright info block.                                               
      |                                                                     
      | Place copyright information at the top of every subsystem in design.
      mask prompts: none "No parameters"
      mask help: Place copyright information at the top of every subsystem in design.
      mask Display:
      | NxtrConf = 'Nexteer Confidential';
      | 
      | sys = bdroot; %handle for the current model ("system")
      | first = get_param(sys,'Created');
      | first = first(end-3:end);  %year is last four digits
      | 
      | last = get_param(sys,'LastModifiedDate');
      | if isempty(last)
      |     last = datestr(now,'yyyy');
      | else
      |     last = last(end-3:end);
      | end
      | 
      | if strcmp(first,last)
      |     fprintf('%s -- Copyright %s Nexteer',NxtrConf,first)
      | else
      |     fprintf('%s -- %s%s- %s Nexteer',NxtrConf,char(169),first,last)
      | end
  Data Store Write : DataStoreWrite  DataStoreName=FastLoopCntrDiagcCfgd
  wires:
  FastLoopCntrDiagcCfgd/1 -> Add/1
  Add/1 -> Data Store Write/1
  Constant/1 -> Add/2

== system ES002A_McuDiagc/McuDiagc/McuDiagcPer1/Increment ISR Based Accumulator/CopyRight2 ==

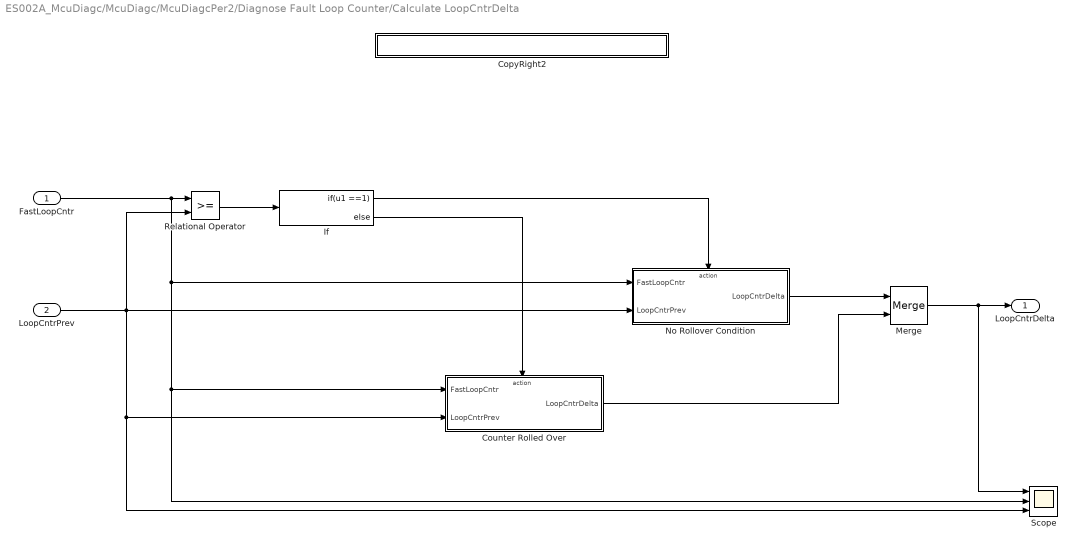
== system ES002A_McuDiagc/McuDiagc/McuDiagcPer2/Diagnose Fault Loop Counter/Calculate LoopCntrDelta ==
  FastLoopCntr : Inport
  LoopCntrPrev : Inport  Port=2
  CopyRight2 : Subsystem  Description=|  mask(Copyright Information){none=on}
      | Copyright info block.                                               
      |                                                                     
      | Place copyright information at the top of every subsystem in design.
      mask prompts: none "No parameters"
      mask help: Place copyright information at the top of every subsystem in design.
      mask Display:
      | NxtrConf = 'Nexteer Confidential';
      | 
      | sys = bdroot; %handle for the current model ("system")
      | first = get_param(sys,'Created');
      | first = first(end-3:end);  %year is last four digits
      | 
      | last = get_param(sys,'LastModifiedDate');
      | if isempty(last)
      |     last = datestr(now,'yyyy');
      | else
      |     last = last(end-3:end);
      | end
      | 
      | if strcmp(first,last)
      |     fprintf('%s -- Copyright %s Nexteer',NxtrConf,first)
      | else
      |     fprintf('%s -- %s%s- %s Nexteer',NxtrConf,char(169),first,last)
      | end
  Counter Rolled Over : Subsystem  TreatAsAtomicUnit=on
  If : If  IfExpression=u1 ==1
  Merge : Merge
  No Rollover Condition : Subsystem  TreatAsAtomicUnit=on
  Relational Operator : RelationalOperator  OutDataTypeStr=boolean
  Scope : Scope  NumInputPorts=3
      settings: YMin=19~0~0  YMax=21~37500~40000
  LoopCntrDelta : Outport
  wires:
  FastLoopCntr/1 -> Scope/2, Counter Rolled Over/1(FastLoopCntr), No Rollover Condition/1(FastLoopCntr), Relational Operator/1
  LoopCntrPrev/1 -> Relational Operator/2, Scope/3, Counter Rolled Over/2(LoopCntrPrev), No Rollover Condition/2(LoopCntrPrev)
  Relational Operator/1 -> If/1
  If/1 -> No Rollover Condition/Action
  If/2 -> Counter Rolled Over/Action
  No Rollover Condition/1(LoopCntrDelta) -> Merge/1
  Counter Rolled Over/1(LoopCntrDelta) -> Merge/2
  Merge/1 -> Scope/1, LoopCntrDelta/1

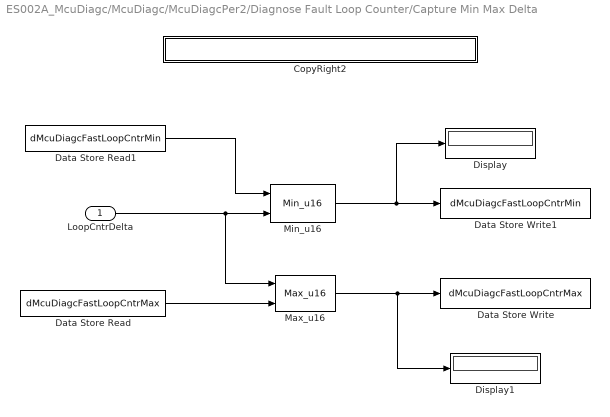
== system ES002A_McuDiagc/McuDiagc/McuDiagcPer2/Diagnose Fault Loop Counter/Capture Min Max Delta ==
  LoopCntrDelta : Inport
  CopyRight2 : Subsystem  Description=|  mask(Copyright Information){none=on}
      | Copyright info block.                                               
      |                                                                     
      | Place copyright information at the top of every subsystem in design.
      mask prompts: none "No parameters"
      mask help: Place copyright information at the top of every subsystem in design.
      mask Display:
      | NxtrConf = 'Nexteer Confidential';
      | 
      | sys = bdroot; %handle for the current model ("system")
      | first = get_param(sys,'Created');
      | first = first(end-3:end);  %year is last four digits
      | 
      | last = get_param(sys,'LastModifiedDate');
      | if isempty(last)
      |     last = datestr(now,'yyyy');
      | else
      |     last = last(end-3:end);
      | end
      | 
      | if strcmp(first,last)
      |     fprintf('%s -- Copyright %s Nexteer',NxtrConf,first)
      | else
      |     fprintf('%s -- %s%s- %s Nexteer',NxtrConf,char(169),first,last)
      | end
  Data Store Read : DataStoreRead  DataStoreName=dMcuDiagcFastLoopCntrMax
  Data Store Read1 : DataStoreRead  DataStoreName=dMcuDiagcFastLoopCntrMin
  Data Store Write : DataStoreWrite  DataStoreName=dMcuDiagcFastLoopCntrMax
  Data Store Write1 : DataStoreWrite  DataStoreName=dMcuDiagcFastLoopCntrMin
  Display : Display
  Display1 : Display
  Max_u16 : NxtrMax/Max_u16  SFunctionSpec=uint16 y1 = Max_u16(uint16 u1, uint16 u2)
      settings: AttributesFormatString=%<Name>
  Min_u16 : NxtrMin/Min_u16  SFunctionSpec=uint16 y1 = Min_u16(uint16 u1, uint16 u2)  ShowSpec=off
      settings: AttributesFormatString=%<Name>
  wires:
  LoopCntrDelta/1 -> Max_u16/1, Min_u16/2
  Max_u16/1 -> Display1/1, Data Store Write/1
  Min_u16/1 -> Display/1, Data Store Write1/1
  Data Store Read/1 -> Max_u16/2
  Data Store Read1/1 -> Min_u16/1

== system ES002A_McuDiagc/McuDiagc/McuDiagcPer2/Diagnose Fault Loop Counter/CopyRight2 ==

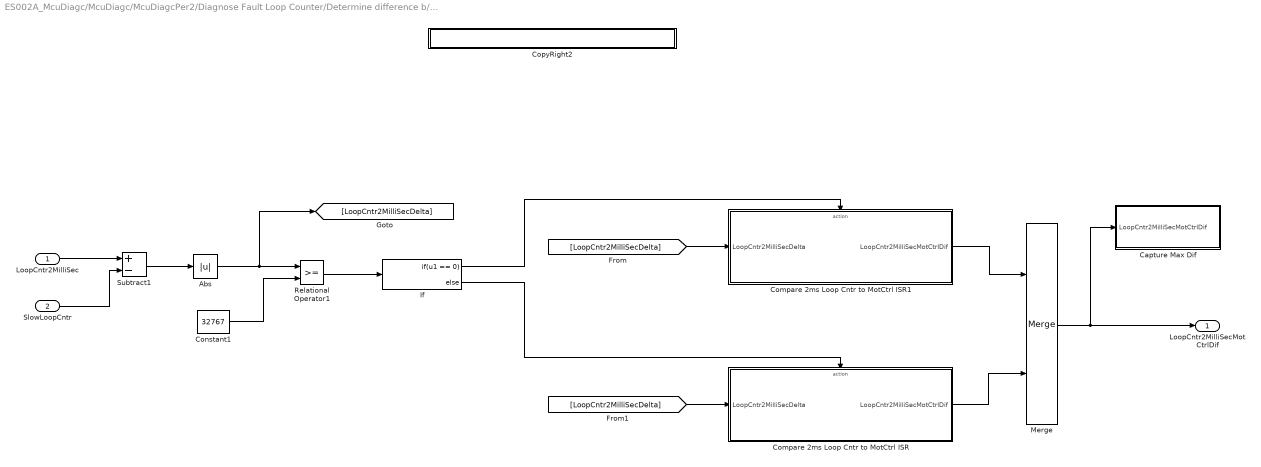
== system ES002A_McuDiagc/McuDiagc/McuDiagcPer2/Diagnose Fault Loop Counter/Determine difference b//w 2ms loop cntr and MotCtrlISR version of 2ms loop cntr ==
  LoopCntr2MilliSec : Inport
  SlowLoopCntr : Inport  Port=2
  Abs : Abs
  Capture Max Dif : Subsystem  TreatAsAtomicUnit=on
  Compare 2ms Loop Cntr to MotCtrl ISR : Subsystem  TreatAsAtomicUnit=on
  Compare 2ms Loop Cntr to MotCtrl ISR1 : Subsystem  TreatAsAtomicUnit=on
  Constant1 : Constant  Description=|  Value=32767  OutDataTypeStr=uint16
      | Half the Data Type max
      | of LoopCnt2MilliSecIntRun 
      | and SlowLoopCntr
      settings: AttributesFormatString=%<Description>
  CopyRight2 : Subsystem  Description=|  mask(Copyright Information){none=on}
      | Copyright info block.                                               
      |                                                                     
      | Place copyright information at the top of every subsystem in design.
      mask prompts: none "No parameters"
      mask help: Place copyright information at the top of every subsystem in design.
      mask Display:
      | NxtrConf = 'Nexteer Confidential';
      | 
      | sys = bdroot; %handle for the current model ("system")
      | first = get_param(sys,'Created');
      | first = first(end-3:end);  %year is last four digits
      | 
      | last = get_param(sys,'LastModifiedDate');
      | if isempty(last)
      |     last = datestr(now,'yyyy');
      | else
      |     last = last(end-3:end);
      | end
      | 
      | if strcmp(first,last)
      |     fprintf('%s -- Copyright %s Nexteer',NxtrConf,first)
      | else
      |     fprintf('%s -- %s%s- %s Nexteer',NxtrConf,char(169),first,last)
      | end
  If : If  IfExpression=u1 == 0
  Merge : Merge
  Relational Operator1 : RelationalOperator  OutDataTypeStr=boolean
  Subtract1 : Sum  Inputs=+-
  LoopCntr2MilliSecMotCtrlDif : Outport
  wires:
  SlowLoopCntr/1 -> Subtract1/2
  LoopCntr2MilliSec/1 -> Subtract1/1
  Subtract1/1 -> Abs/1
  Abs/1 -> [LoopCntr2MilliSecDelta], Relational Operator1/1
  Compare 2ms Loop Cntr to MotCtrl ISR1/1(LoopCntr2MilliSecMotCtrlDif) -> Merge/1
  Compare 2ms Loop Cntr to MotCtrl ISR/1(LoopCntr2MilliSecMotCtrlDif) -> Merge/2
  [LoopCntr2MilliSecDelta] -> Compare 2ms Loop Cntr to MotCtrl ISR/1(LoopCntr2MilliSecDelta)
  [LoopCntr2MilliSecDelta] -> Compare 2ms Loop Cntr to MotCtrl ISR1/1(LoopCntr2MilliSecDelta)
  Merge/1 -> Capture Max Dif/1(LoopCntr2MilliSecMotCtrlDif), LoopCntr2MilliSecMotCtrlDif/1
  If/1 -> Compare 2ms Loop Cntr to MotCtrl ISR1/Action
  If/2 -> Compare 2ms Loop Cntr to MotCtrl ISR/Action
  Constant1/1 -> Relational Operator1/2
  Relational Operator1/1 -> If/1

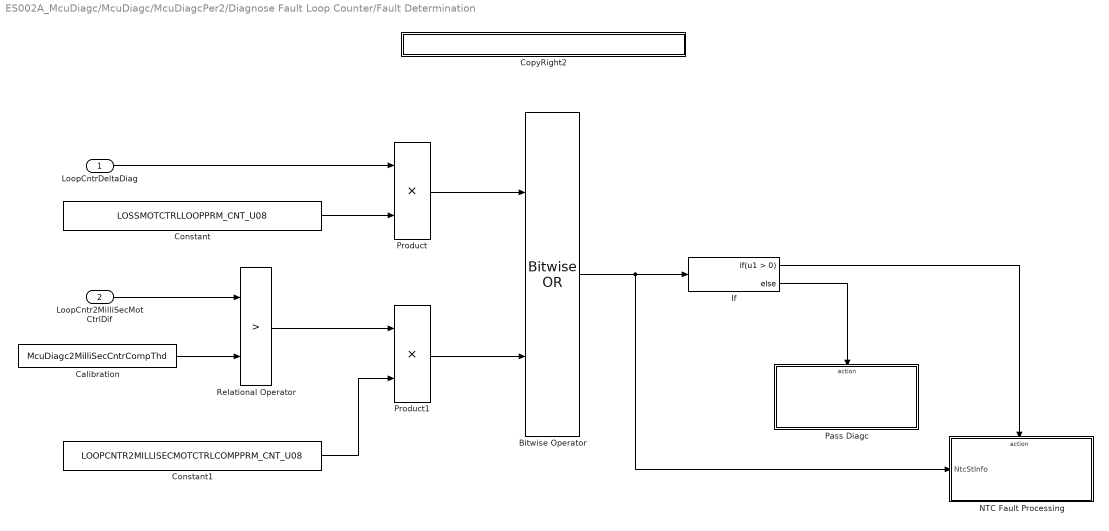
== system ES002A_McuDiagc/McuDiagc/McuDiagcPer2/Diagnose Fault Loop Counter/Fault Determination ==
  LoopCntrDeltaDiag : Inport
  LoopCntr2MilliSecMotCtrlDif : Inport  Port=2
  Bitwise Operator : simulink/Logic and Bit Operations/Bitwise Operator  logicop=OR  UseBitMask=off  NumInputPorts=2  BitMask=bin2dec('11011001')  BitMaskRealWorld=Stored Integer
  Calibration : Constant  Value=McuDiagc2MilliSecCntrCompThd
  Constant : Constant  Value=LOSSMOTCTRLLOOPPRM_CNT_U08  OutDataTypeStr=uint8
  Constant1 : Constant  Value=LOOPCNTR2MILLISECMOTCTRLCOMPPRM_CNT_U08  OutDataTypeStr=uint8
  CopyRight2 : Subsystem  Description=|  mask(Copyright Information){none=on}
      | Copyright info block.                                               
      |                                                                     
      | Place copyright information at the top of every subsystem in design.
      mask prompts: none "No parameters"
      mask help: Place copyright information at the top of every subsystem in design.
      mask Display:
      | NxtrConf = 'Nexteer Confidential';
      | 
      | sys = bdroot; %handle for the current model ("system")
      | first = get_param(sys,'Created');
      | first = first(end-3:end);  %year is last four digits
      | 
      | last = get_param(sys,'LastModifiedDate');
      | if isempty(last)
      |     last = datestr(now,'yyyy');
      | else
      |     last = last(end-3:end);
      | end
      | 
      | if strcmp(first,last)
      |     fprintf('%s -- Copyright %s Nexteer',NxtrConf,first)
      | else
      |     fprintf('%s -- %s%s- %s Nexteer',NxtrConf,char(169),first,last)
      | end
  If : If
  NTC Fault Processing : Subsystem  RequirementInfo="{'linktype_rmi_doors' '00010239 (/ESG Group/FDD Module Requirements/EA4 Specific/ES002A_McuDiagc)' '#ES002A_22' 'true' 'REQ:  ES002A_22' '' ; 'linktype_rmi_doors' '00010239 (/ESG Group/FDD Module Requirements/EA4 Specific/ES002A_McuDiagc)' '#ES002A_31' 'true' 'REQ:  ES002A_31' '' ; 'linktype_rmi_doors' '00010239 (/ESG Group/FDD Module Requirements/EA4 Specific/ES002A_McuDiagc)' '#ES002A_22' 'true' 'REQ:ES002A_22' '' } %GIDa_09aba030_ff97_4621_8436_dd77fed4eeff"  TreatAsAtomicUnit=on
  Pass Diagc : Subsystem  RequirementInfo={'linktype_rmi_doors' '00010239 (/ESG Group/FDD Module Requirements/EA4 Specific/ES002A_McuDiagc)' '#ES002A_22' 'true' 'REQ:ES002A_22' '' ; 'linktype_rmi_doors' '00010239 (/ESG Group/FDD Module Requirements/EA4 Specific/ES002A_McuDiagc)' '#ES002A_31' 'true' 'REQ:ES002A_31' '' } %GIDa_d7b96987_3a81_48c0_aff1_0aaf4d523386  TreatAsAtomicUnit=on
  Product : Product
  Product1 : Product
  Relational Operator : RelationalOperator  RequirementInfo="{'linktype_rmi_doors' '00010239 (/ESG Group/FDD Module Requirements/EA4 Specific/ES002A_McuDiagc)' '#ES002A_65' 'true' 'REQ:  ES002A_65' '' } %GIDa_72b7605d_75e6_4fe8_978d_249daf62e5fe"  Operator=>  OutDataTypeStr=boolean
  wires:
  LoopCntr2MilliSecMotCtrlDif/1 -> Relational Operator/1
  Calibration/1 -> Relational Operator/2
  Product/1 -> Bitwise Operator/1
  Product1/1 -> Bitwise Operator/2
  Relational Operator/1 -> Product1/1
  LoopCntrDeltaDiag/1 -> Product/1
  Bitwise Operator/1 -> NTC Fault Processing/1(NtcStInfo), If/1
  If/1 -> NTC Fault Processing/Action
  If/2 -> Pass Diagc/Action
  Constant/1 -> Product/2
  Constant1/1 -> Product1/2

== system ES002A_McuDiagc/McuDiagc/McuDiagcPer2/Diagnose Fault Loop Counter/Motor Control Loop counter diagnosis ==
  LoopCntrDelta : Inport
  Constant : Constant  Value=FASTLOOPCNTRMAX_CNT_U08
  Constant1 : Constant  Value=FASTLOOPCNTRMIN_CNT_U08
  CopyRight2 : Subsystem  Description=|  mask(Copyright Information){none=on}
      | Copyright info block.                                               
      |                                                                     
      | Place copyright information at the top of every subsystem in design.
      mask prompts: none "No parameters"
      mask help: Place copyright information at the top of every subsystem in design.
      mask Display:
      | NxtrConf = 'Nexteer Confidential';
      | 
      | sys = bdroot; %handle for the current model ("system")
      | first = get_param(sys,'Created');
      | first = first(end-3:end);  %year is last four digits
      | 
      | last = get_param(sys,'LastModifiedDate');
      | if isempty(last)
      |     last = datestr(now,'yyyy');
      | else
      |     last = last(end-3:end);
      | end
      | 
      | if strcmp(first,last)
      |     fprintf('%s -- Copyright %s Nexteer',NxtrConf,first)
      | else
      |     fprintf('%s -- %s%s- %s Nexteer',NxtrConf,char(169),first,last)
      | end
  Logical Operator : Logic  Operator=OR  AllPortsSameDT=off  OutDataTypeStr=boolean
  Relational Operator : RelationalOperator  RequirementInfo="{'linktype_rmi_doors' '00010239 (/ESG Group/FDD Module Requirements/EA4 Specific/ES002A_McuDiagc)' '#ES002A_65' 'true' 'REQ:  ES002A_65' '' } %GIDa_fe65c9c6_4bda_46e5_b409_139105a12e8d"  Operator=>  OutDataTypeStr=boolean
  Relational Operator1 : RelationalOperator  RequirementInfo="{'linktype_rmi_doors' '00010239 (/ESG Group/FDD Module Requirements/EA4 Specific/ES002A_McuDiagc)' '#ES002A_66' 'true' 'REQ:  ES002A_66' '' } %GIDa_2b13d053_9bbb_44ca_8ecb_c69241b77ad6"  Operator=<  OutDataTypeStr=boolean
  LoopCntrDeltaDiag : Outport
  wires:
  LoopCntrDelta/1 -> Relational Operator1/1, Relational Operator/1
  Constant1/1 -> Relational Operator1/2
  Constant/1 -> Relational Operator/2
  Relational Operator/1 -> Logical Operator/1
  Relational Operator1/1 -> Logical Operator/2
  Logical Operator/1 -> LoopCntrDeltaDiag/1

== system ES002A_McuDiagc/McuDiagc/McuDiagcPer2/Increment 2ms loop  counter/CopyRight2 ==

== system ES002A_McuDiagc/McuDiagc/McuDiagcPer2/Pass Loop Counter Diagc/CopyRight2 ==

== system ES002A_McuDiagc/McuDiagc/McuDiagcPer2/Diagnose Fault Loop Counter/Calculate LoopCntrDelta/CopyRight2 ==
